simulink model "GFLIB_IntegratorTR_BAM_F32"  (Simulink 7.3)
settings: Solver=ode45  StartTime=0.0  StopTime=10.0  RelTol=1e-3
undefined symbols (not defined in the file): f32C1, u16NShift
settings Model: Creator=RE004C  LastModifiedBy=RE004C
settings HardwareCC: ProdIntDivRoundTo=Zero  ProdEndianess=BigEndian  ProdHWDeviceType=Freescale->32-bit PowerPC

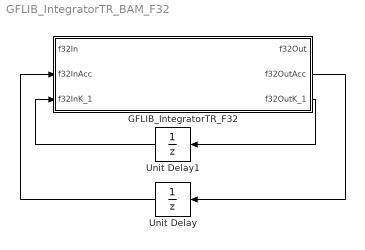
== system GFLIB_IntegratorTR_BAM_F32 ==
  GFLIB_IntegratorTR_F32 : Subsystem  mask(GFLIB_IntegratorTR_F32){f32C1=f32C1, u16NShift=u16NShift}
      mask help: Bit accurate model of discrete trapezoidal integrator. All parameters as well as input and output are full float range.
      mask init:
      | pos = get_param(gcb, 'Position');width = pos(3) - pos(1); height = pos(4) - pos(2);tX=width/2;tY=height*0.9;
      mask Display:
      | color('black');
      | port_label('input',1,'f32In');
      | port_label('input',2,'f32InAcc');
      | port_label('input',3,'f32InK_1');
      | port_label('output',1,'f32Out');
      | port_label('output',2,'f32OutAcc');
      | port_label('output',3,'f32OutK_1');
      | color('black');
      | disp('GFLIB_IntegratorTR_F32');
      | color('blue');
      | text(tX,tY, 'BAM', 'horizontalAlignment', 'center');
  Unit Delay : UnitDelay  SampleTime=-1
  Unit Delay1 : UnitDelay  SampleTime=-1
  wires:
  GFLIB_IntegratorTR_F32/2(f32OutAcc) -> Unit Delay/1
  Unit Delay/1 -> GFLIB_IntegratorTR_F32/2(f32InAcc)
  GFLIB_IntegratorTR_F32/3(f32OutK_1) -> Unit Delay1/1
  Unit Delay1/1 -> GFLIB_IntegratorTR_F32/3(f32InK_1)

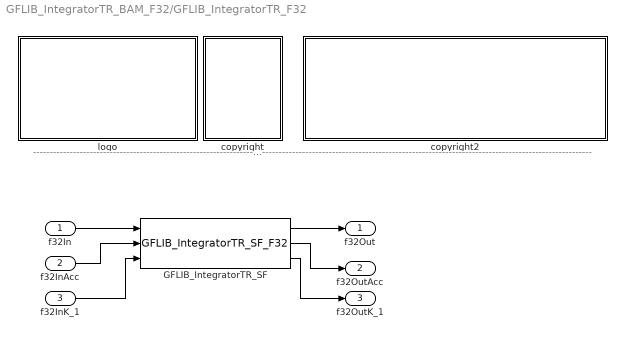
== system GFLIB_IntegratorTR_BAM_F32/GFLIB_IntegratorTR_F32 ==
  note: ---------------------------------------------------------------------------------------------------------------------------------------------------------------------------------------------------
  f32In : Inport  OutDataType=fixdt(1, 16)  OutScaling=2^0
  f32InAcc : Inport  Port=2  OutDataType=fixdt(1, 16)  OutScaling=2^0
  f32InK_1 : Inport  Port=3  OutDataType=fixdt(1, 16)  OutScaling=2^0
  GFLIB_IntegratorTR_SF : S-Function  FunctionName=GFLIB_IntegratorTR_SF_F32  Parameters=f32C1,u16NShift  EnableBusSupport=off
  copyright : Subsystem
      mask Display: text(10,90,'FILE:');text(10,75,'DESRIPTION:')text(10,60,'COPYRIGHT:')text(10,45,'VERSION:')text(10,30,'DATE:')
  copyright2 : Subsystem
      mask Display: text(10,90,'GFLIB_IntegratorTR_BAM_F32.mdl');text(10,75,'Discrete integrator transformed from linear model using Billinear (trapezoidal) transformation.');text(10,60,'Freescale')text(10,45,'0.1');text(10,30,'16-Jan-2012');
  logo : Subsystem
      mask Display: image(imread('logo.jpg'))
  f32Out : Outport  OutDataType=fixdt(1, 16)  OutScaling=2^0
  f32OutAcc : Outport  Port=2  OutDataType=fixdt(1, 16)  OutScaling=2^0
  f32OutK_1 : Outport  Port=3  OutDataType=fixdt(1, 16)  OutScaling=2^0
  wires:
  f32In/1 -> GFLIB_IntegratorTR_SF/1
  GFLIB_IntegratorTR_SF/1 -> f32Out/1
  GFLIB_IntegratorTR_SF/2 -> f32OutAcc/1
  GFLIB_IntegratorTR_SF/3 -> f32OutK_1/1
  f32InAcc/1 -> GFLIB_IntegratorTR_SF/2
  f32InK_1/1 -> GFLIB_IntegratorTR_SF/3

== system GFLIB_IntegratorTR_BAM_F32/GFLIB_IntegratorTR_F32/copyright ==

== system GFLIB_IntegratorTR_BAM_F32/GFLIB_IntegratorTR_F32/copyright2 ==

== system GFLIB_IntegratorTR_BAM_F32/GFLIB_IntegratorTR_F32/logo ==
